simulink model "singalAriClinder"  (R2018a)
settings: Solver=FixedStepAuto  StartTime=0.0  StopTime=30.0  FixedStep=1  RelTol=1e-3
settings Model: Creator=wangmt  LastModifiedBy=wangmt

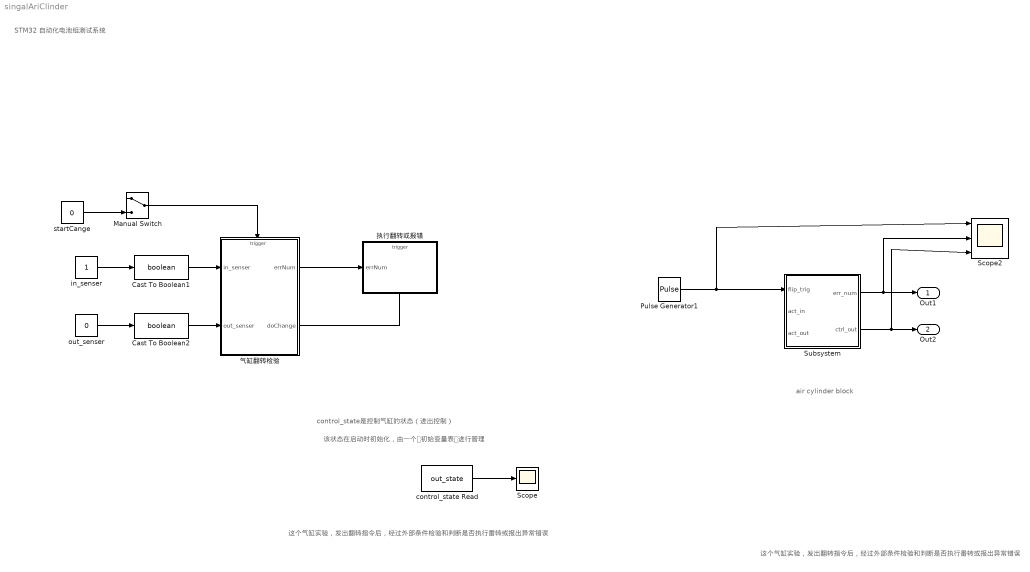
== system singalAriClinder ==
  note: air cylinder block
  note: 该状态在启动时初始化，由一个〈初始变量表〉进行管理
  note: control_state是控制气缸的状态（进出控制）
  note: 这个气缸实验，发出翻转指令后，经过外部条件检验和判断是否执行番转或报出异常错误
  note: STM32
      | 自动化电池组测试系统
  note: 这个气缸实验，发出翻转指令后，经过外部条件检验和判断是否执行番转或报出异常错误
  Cast To Boolean1 : DataTypeConversion  OutDataTypeStr=boolean
  Cast To Boolean2 : DataTypeConversion  OutDataTypeStr=boolean
  Manual Switch : ManualSwitch
  Pulse Generator1 : DiscretePulseGenerator  PulseType=Time based  PulseWidth=50
  Scope : Scope
  Scope2 : Scope  NumInputPorts=3
  Subsystem : Subsystem
  control_state Read : DataStoreRead  DataStoreName=out_state
  in_senser : Constant
  out_senser : Constant  Value=0
  "startCange " : Constant  Value=0
  执行翻转或报错 : Stateflow chart  TreatAsAtomicUnit=on
  气缸翻转检验 : Stateflow chart  TreatAsAtomicUnit=on
  Out1 : Outport
  Out2 : Outport  Port=2
  wires:
  out_senser/1 -> Cast To Boolean2/1
  in_senser/1 -> Cast To Boolean1/1
  气缸翻转检验/1(errNum) -> 执行翻转或报错/1(errNum)
  Cast To Boolean1/1 -> 气缸翻转检验/1(in_senser)
  Cast To Boolean2/1 -> 气缸翻转检验/2(out_senser)
  control_state Read/1 -> Scope/1
  Manual Switch/1 -> 气缸翻转检验/Trigger
  "startCange "/1 -> Manual Switch/2
  气缸翻转检验/2(doChange) -> 执行翻转或报错/Trigger
  Subsystem/1(err_num) -> Scope2/2, Out1/1
  Pulse Generator1/1 -> Scope2/1, Subsystem/1(flip_trig)
  Subsystem/2(ctrl_out) -> Scope2/3, Out2/1

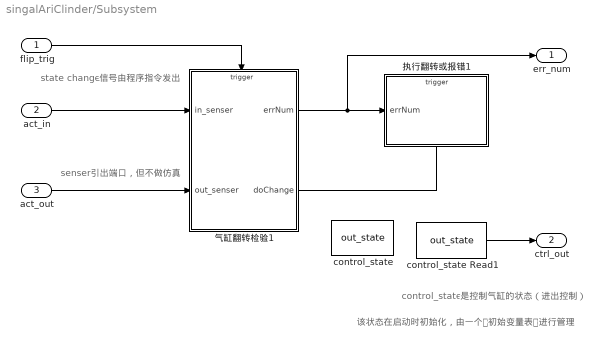
== system singalAriClinder/Subsystem ==
  note: senser引出端口，但不做仿真
  note: state change信号由程序指令发出
  note: 该状态在启动时初始化，由一个〈初始变量表〉进行管理
  note: control_state是控制气缸的状态（进出控制）
  flip_trig : Inport
  act_in : Inport  Port=2
  act_out : Inport  Port=3
  control_state : DataStoreMemory  DataStoreName=out_state  ReadBeforeWriteMsg=warning  WriteAfterWriteMsg=warning  WriteAfterReadMsg=warning  InitialValue=false  ShowAdditionalParam=off  OutDataTypeStr=boolean
  control_state Read1 : DataStoreRead  DataStoreName=out_state
  执行翻转或报错1 : Stateflow chart  TreatAsAtomicUnit=on
  气缸翻转检验1 : Stateflow chart  TreatAsAtomicUnit=on
  err_num : Outport
  ctrl_out : Outport  Port=2
  wires:
  control_state Read1/1 -> ctrl_out/1
  act_out/1 -> 气缸翻转检验1/2(out_senser)
  气缸翻转检验1/2(doChange) -> 执行翻转或报错1/Trigger
  flip_trig/1 -> 气缸翻转检验1/Trigger
  气缸翻转检验1/1(errNum) -> err_num/1, 执行翻转或报错1/1(errNum)
  act_in/1 -> 气缸翻转检验1/1(in_senser)

== stateflow chart singalAriClinder/气缸翻转检验 ==
  note: startChange有效，再把startChange转发出去
  note: 气缸交换状态真值表
      | 返回是否可以执行转换
  note: 一个气缸动作的相关参数：
      | 输入有3个：（来自外设的GPIO）
      | cyl_outsta.        当前的气缸状态(是否在输出状态）     --- 1个
      | in_sen--out_sen. 当前进出的感应头状态  --- 2个
      |
      | 输出有1个
      | error. 错误 --- 1个
  (default) -> (junction 21) : startChange{errNum =CylinderCanChange(out_state, in_senser, out_senser);}
  data: cyl_outSta function_input boolean; in_sen function_input boolean; out_sen function_input boolean; error function_output double; errNum output double =5; in_senser input; out_senser input; out_state data_store_memory
  events: startChange input EITHER_EDGE_EVENT; doChange output EITHER_EDGE_EVENT
  function error=CylinderCanChange(cyl_outSta,in_sen,out_sen):
    | function error=CylinderCanChange(cyl_outSta,in_sen,out_sen)
    | 
    | aVarTruthTableCondition_1 = false;
    | aVarTruthTableCondition_2 = false;
    | aVarTruthTableCondition_3 = false;
    | 
    | 
    | % 气缸在伸出状态
    | 
    | aVarTruthTableCondition_1 = logical(cyl_outSta==true);
    | 
    | % 缩进传感器点亮
    | 
    | aVarTruthTableCondition_2 = logical(in_sen==true);
    | 
    | % 伸出传感器点亮
    | 
    | aVarTruthTableCondition_3 = logical(out_sen==true);
    | 
    | if (aVarTruthTableCondition_1 && ~aVarTruthTableCondition_2 && ~aVarTruthTableCondition_3)
    |     no_err1();
    | elseif (~aVarTruthTableCondition_1 && ~aVarTruthTableCondition_2 && ~aVarTruthTableCondition_3)
    |     no_err1();
    | elseif (aVarTruthTableCondition_1 && aVarTruthTableCondition_2 && aVarTruthTableCondition_3)
    |     err2();
    | elseif (~aVarTruthTableCondition_1 && aVarTruthTableCondition_2 && aVarTruthTableCondition_3)
    |     err2();
    | elseif (aVarTruthTableCondition_1 && ~aVarTruthTableCondition_2 && aVarTruthTableCondition_3)
    |     no_err();
    | elseif (aVarTruthTableCondition_1 && aVarTruthTableCondition_2 && ~aVarTruthTableCondition_3)
    |     err1();
    | elseif (~aVarTruthTableCondition_1 && aVarTruthTableCondition_2 && ~aVarTruthTableCondition_3)
    |     no_err();
    | else % Default
    |     err1();
    | end
    | 
    | function no_err()
    | 
    | % 没有错误(sta/sen一致）
    | 
    | error=0;
    | 
    | function err1()
    | 
    | % 错误1(sta/sen不一致，传感器反了）
    | 
    | error=1;
    | 
    | function err2()
    | 
    | % 错误2(两sen状态一起为ON，传感器可能故障）
    | 
    | error=2;
    | 
    | function no_err1()
    | 
    | % 没有错误(sta/sen一致为OFF，case1: 未装传感器；case2: 气缸行进中）
    | % 正常情况下，执行气缸翻转遇不到case2. 故此情况当作OK，并设开始转换到感应信号检测不到的超时判断。（若无传感器不做判断）
    | 
    | error=-2;

== stateflow chart singalAriClinder/Subsystem/执行翻转或报错1 ==
  note: 路径2,改变当前的out_state
  (default) -> (junction 7) : doChange
  (junction 7) -> (junction 8) [order 1] : [errNum>0]
  (junction 7) -> (junction 9) [order 2] : {out_state=~out_state;}
  (junction 8) -> (junction 10) : {out_state=out_state;}
  (junction 10) -> (junction 9)
  (junction 9) -> (junction 11)
  data: errNum input; out_state data_store_memory
  events: doChange input EITHER_EDGE_EVENT

== stateflow chart singalAriClinder/执行翻转或报错 ==
  note: 路径2,改变当前的out_state
  (default) -> (junction 7) : doChange
  (junction 7) -> (junction 8) [order 1] : [errNum>0]
  (junction 7) -> (junction 9) [order 2] : {out_state=~out_state;}
  (junction 8) -> (junction 10) : {out_state=out_state;}
  (junction 10) -> (junction 9)
  (junction 9) -> (junction 11)
  data: errNum input; out_state data_store_memory
  events: doChange input EITHER_EDGE_EVENT

== stateflow chart singalAriClinder/Subsystem/气缸翻转检验1 ==
  note: startChange有效，再把startChange转发出去
  note: 气缸交换状态真值表
      | 返回是否可以执行转换
  note: 一个气缸动作的相关参数：
      | 输入有3个：（来自外设的GPIO）
      | cyl_outsta.        当前的气缸状态(是否在输出状态）     --- 1个
      | in_sen--out_sen. 当前进出的感应头状态  --- 2个
      |
      | 输出有1个
      | error. 错误 --- 1个
  (default) -> (junction 21) : startChange{errNum =CylinderCanChange(out_state, in_senser, out_senser);}
  data: cyl_outSta function_input boolean; in_sen function_input boolean; out_sen function_input boolean; error function_output double; errNum output double =5; in_senser input; out_senser input; out_state data_store_memory
  events: startChange input EITHER_EDGE_EVENT; doChange output EITHER_EDGE_EVENT
  function error=CylinderCanChange(cyl_outSta,in_sen,out_sen):
    | function error=CylinderCanChange(cyl_outSta,in_sen,out_sen)
    | 
    | aVarTruthTableCondition_1 = false;
    | aVarTruthTableCondition_2 = false;
    | aVarTruthTableCondition_3 = false;
    | 
    | 
    | % 气缸在伸出状态
    | 
    | aVarTruthTableCondition_1 = logical(cyl_outSta==true);
    | 
    | % 缩进传感器点亮
    | 
    | aVarTruthTableCondition_2 = logical(in_sen==true);
    | 
    | % 伸出传感器点亮
    | 
    | aVarTruthTableCondition_3 = logical(out_sen==true);
    | 
    | if (aVarTruthTableCondition_1 && ~aVarTruthTableCondition_2 && ~aVarTruthTableCondition_3)
    |     no_err1();
    | elseif (~aVarTruthTableCondition_1 && ~aVarTruthTableCondition_2 && ~aVarTruthTableCondition_3)
    |     no_err1();
    | elseif (aVarTruthTableCondition_1 && aVarTruthTableCondition_2 && aVarTruthTableCondition_3)
    |     err2();
    | elseif (~aVarTruthTableCondition_1 && aVarTruthTableCondition_2 && aVarTruthTableCondition_3)
    |     err2();
    | elseif (aVarTruthTableCondition_1 && ~aVarTruthTableCondition_2 && aVarTruthTableCondition_3)
    |     no_err();
    | elseif (aVarTruthTableCondition_1 && aVarTruthTableCondition_2 && ~aVarTruthTableCondition_3)
    |     err1();
    | elseif (~aVarTruthTableCondition_1 && aVarTruthTableCondition_2 && ~aVarTruthTableCondition_3)
    |     no_err();
    | else % Default
    |     err1();
    | end
    | 
    | function no_err()
    | 
    | % 没有错误(sta/sen一致）
    | 
    | error=0;
    | 
    | function err1()
    | 
    | % 错误1(sta/sen不一致，传感器反了）
    | 
    | error=1;
    | 
    | function err2()
    | 
    | % 错误2(两sen状态一起为ON，传感器可能故障）
    | 
    | error=2;
    | 
    | function no_err1()
    | 
    | % 没有错误(sta/sen一致为OFF，case1: 未装传感器；case2: 气缸行进中）
    | % 正常情况下，执行气缸翻转遇不到case2. 故此情况当作OK，并设开始转换到感应信号检测不到的超时判断。（若无传感器不做判断）
    | 
    | error=-2;
